simulink model "airspeed_from_throttle_loop"  (Simulink 8.0)
settings: Solver=ode45  StartTime=0.0  StopTime=100  RelTol=1e-3
values from neighbouring files (symbols this model uses):
  a_Vt1 = den(2)    [computeGains.m]
  a_Vt2 = num(2)    [computeGains.m]
undefined symbols (not defined in the file or in its folder): P
settings Model: Creator=beard  LastModifiedBy=Gary
settings DataIOCC: SignalLoggingSaveFormat=ModelDataLogs
settings DebuggingCC: FcnCallInpInsideContextMsg=UseLocalSettings  StrictBusMsg=Warning
settings GRTTargetCC: CombineOutputUpdateFcns=off  GRTInterface=on

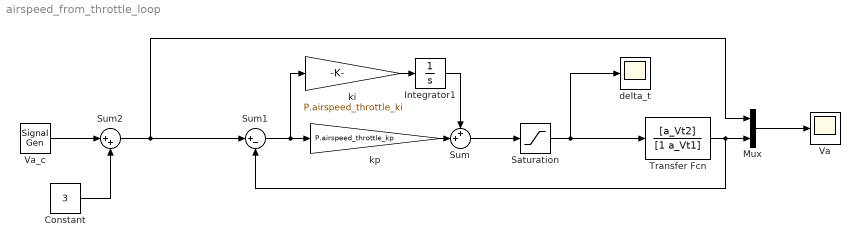
== system airspeed_from_throttle_loop ==
  Constant : Constant  Value=3
  Integrator1 : Integrator
  Mux : Mux  Inputs=2
  Saturation : Saturate  UpperLimit=1  LowerLimit=0
  Sum : Sum  Inputs=++|
  Sum1 : Sum  Inputs=|+-
  Sum2 : Sum  Inputs=|++
  Transfer Fcn : TransferFcn  Numerator=[a_Vt2]  Denominator=[1 a_Vt1]
  Va : Scope
      settings: TimeRange=100  YMin=-3  YMax=3
  Va_c : SignalGenerator  WaveForm=square  Amplitude=2  Frequency=.02
  delta_t : Scope
      settings: TimeRange=100  YMin=-3  YMax=3
  ki : Gain  Gain=P.airspeed_throttle_ki
  kp : Gain  Gain=P.airspeed_throttle_kp
  wires:
  Sum/1 -> Saturation/1
  kp/1 -> Sum/2
  Sum1/1 -> kp/1, ki/1
  ki/1 -> Integrator1/1
  Integrator1/1 -> Sum/1
  Mux/1 -> Va/1
  Transfer Fcn/1 -> Mux/2, Sum1/2
  Saturation/1 -> Transfer Fcn/1, delta_t/1
  Va_c/1 -> Sum2/1
  Constant/1 -> Sum2/2
  Sum2/1 -> Sum1/1, Mux/1
